simulink model "mainLinR2"  (R2017a)
settings: Solver=ode45  StartTime=0.0  StopTime=Tsim  RelTol=1e-3
values from neighbouring files (symbols this model uses):
  D = C2.Kd    [mainRun.m]
  F = -2    [mainRun.m]
  g = .5    (= 0.5)    [mainRun.m]
  Gamma = 10*eye(4)    [mainRun.m]
  I = C2.Ki    [mainRun.m]
  Kr0 = 0    [mainRun.m]
  Kx0 = 0    [mainRun.m]
  N = 2    [ident_wynik.m]    (also in mainRun.m = 1/C2.Tf; odp_czas.m = size(wyjscia,2); wykresyBode.m = length(modele))
  NAref = mrac.A    [mainRun.m]
  NBref = mrac.B    [mainRun.m]
  NCref = mrac.C    [mainRun.m]
  Nxref0 = zeros(2,1)    [mainRun.m]
  p0 = 1    [mainRun.m]
  phi0 = zeros(4,1)    [mainRun.m]
  PPid = C2.Kp    [mainRun.m]
  szum = 2e-4    (= 0.0002)    [mainRun.m]
  Th0 = zeros(4,1)    [mainRun.m]
  w10 = 0    [mainRun.m]
  w20 = 0    [mainRun.m]
  Xref0 = 0    [mainRun.m]
undefined symbols (not defined in the file or in its folder): GammaR, GammaX, P
libraries: bloki_pomocnicze x12, simulink x2, dspstat3 x2
settings Model: Creator=Piotr  LastModifiedBy=Piotr
settings SolverCC: ZeroCrossAlgorithm=Adaptive
settings OptimizationCC: EfficientFloat2IntCast=on
settings DebuggingCC: MaskedZcDiagnostic=none  IgnoredZcDiagnostic=none

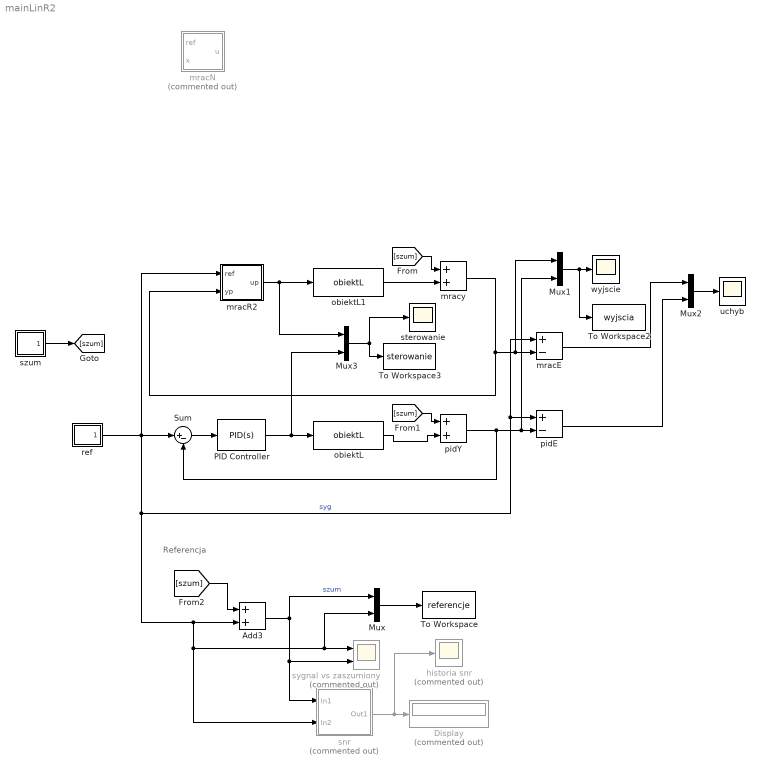
== system mainLinR2 ==
  note: Referencja
  Add3 : Sum
  Display : Display  Commented=on
  Mux{,1..3} (4 alike) : Mux  Inputs=2
  PID Controller : simulink/Continuous/PID Controller  Controller=PID  TimeDomain=Continuous-time  SampleTime=-1  IntegratorMethod=Forward Euler  FilterMethod=Forward Euler  Form=Parallel  UseFilter=on  ControllerParametersSource=internal  P=PPid  I=I  D=D  N=N  InitialConditionSource=internal  InitialConditionForIntegrator=0  InitialConditionForFilter=0  ExternalReset=none  LimitOutput=off  UpperSaturationLimit=1e6  LowerSaturationLimit=-1e6  LinearizeAsGain=on  AntiWindupMode=none  Kb=1  TrackingMode=off  Kt=1  PParamMin=[]  PParamMax=[]  IParamMin=[]  IParamMax=[]  DParamMin=[]  DParamMax=[]  NParamMin=[]  NParamMax=[]  KbParamMin=[]  KbParamMax=[]  KtParamMin=[]  KtParamMax=[]  POutMin=[]  POutMax=[]  IOutMin=[]  IOutMax=[]  DOutMin=[]  DOutMax=[]  NOutMin=[]  NOutMax=[]  KbOutMin=[]  KbOutMax=[]  KtOutMin=[]  KtOutMax=[]  IntegratorOutMin=[]  IntegratorOutMax=[]  FilterOutMin=[]  FilterOutMax=[]  SumOutMin=[]  SumOutMax=[]  SumI1OutMin=[]  SumI1OutMax=[]  SumI2OutMin=[]  SumI2OutMax=[]  SumI3OutMin=[]  SumI3OutMax=[]  SumDOutMin=[]  SumDOutMax=[]  SaturationOutMin=[]  SaturationOutMax=[]  IntegratorContinuousStateAttributes=''  IntegratorStateMustResolveToSignalObject=off  IntegratorRTWStateStorageClass=Auto  FilterContinuousStateAttributes=''  FilterStateMustResolveToSignalObject=off  FilterRTWStateStorageClass=Auto  DifferentiatorICPrevScaledInput=0  DifferentiatorOutMin=[]  DifferentiatorOutMax=[]  InitialConditionSetting=State (most efficient)
  Sum : Sum  Inputs=|+-
  To Workspace : ToWorkspace  VariableName=referencje  SampleTime=-1
  To Workspace2 : ToWorkspace  VariableName=wyjscia  SampleTime=-1
  To Workspace3 : ToWorkspace  VariableName=sterowanie  SampleTime=-1
  historia snr : Scope  Commented=on
  mracE : Sum  Inputs=+-
  mracN : Subsystem  Commented=on
  mracR2 : Subsystem  AncestorBlock=bloki_pomocnicze/mracR2
  mracy : Sum
  obiektL : bloki_pomocnicze/obiektL  SystemSampleTime=-1
  obiektL1 : bloki_pomocnicze/obiektL  SystemSampleTime=-1
  pidE : Sum  Inputs=+-
  pidY : Sum
  ref : Subsystem
  snr : Subsystem  Commented=on
  sterowanie : Scope
  sygnal vs zaszumiony : Scope  Commented=on  NumInputPorts=2
  szum : Subsystem
  uchyb : Scope
  wyjscie : Scope
  wires:
  PID Controller/1 -> Mux3/2, obiektL/1
  Sum/1 -> PID Controller/1
  pidY/1 -> Sum/2, Mux1/2, pidE/2
  mracy/1 -> mracR2/2(yp), Mux1/1, mracE/2
  mracE/1 -> Mux2/1
  pidE/1 -> Mux2/2
  Add3/1 -> snr/1(In1), sygnal vs zaszumiony/2, Mux/1  "szum"
  snr/1(Out1) -> historia snr/1, Display/1
  szum/1(Out1) -> [szum]
  obiektL1/1 -> mracy/2
  [szum] -> mracy/1
  obiektL/1 -> pidY/2
  [szum] -> pidY/1
  [szum] -> Add3/1
  ref/1(Out1) -> mracR2/1(ref), mracE/1, pidE/1, Add3/2, snr/2(In2), sygnal vs zaszumiony/1, Mux/2, Sum/1  "syg"
  Mux/1 -> To Workspace/1
  Mux1/1 -> To Workspace2/1, wyjscie/1
  Mux2/1 -> uchyb/1
  Mux3/1 -> To Workspace3/1, sterowanie/1
  mracR2/1(up) -> Mux3/1, obiektL1/1

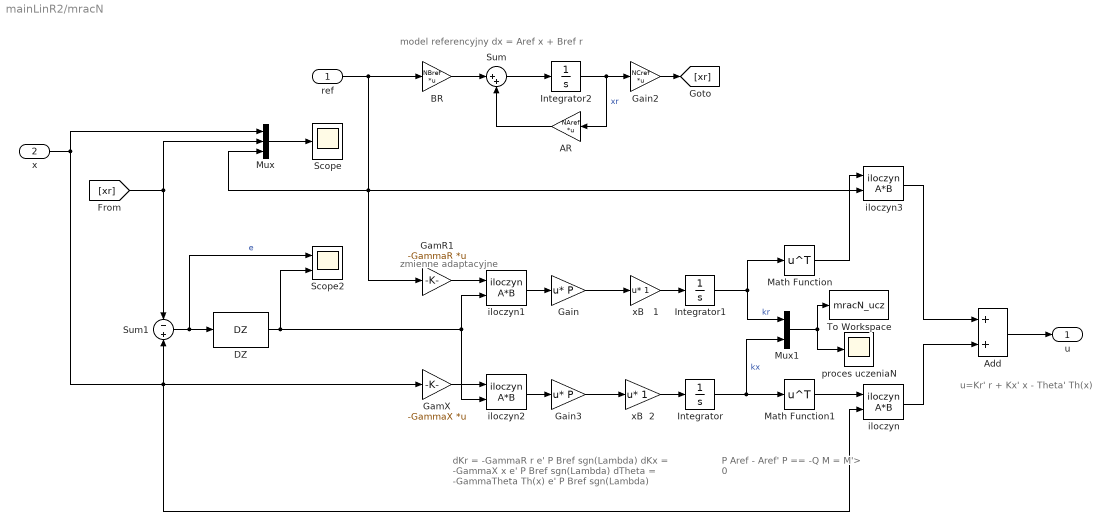
== system mainLinR2/mracN ==
  note: P Aref - Aref' P == -Q
      |
      | M = M'> 0
  note: dKr = -GammaR r e' P Bref sgn(Lambda)
      | dKx = -GammaX x e' P Bref sgn(Lambda)
      | dTheta = -GammaTheta Th(x) e' P Bref sgn(Lambda)
  note: zmienne adaptacyjne
  note: model referencyjny dx = Aref x + Bref r
  note: u=Kr' r + Kx' x - Theta' Th(x)
  ref : Inport
  x : Inport  Port=2
  AR : Gain  Gain=NAref  Multiplication=Matrix(K*u)
  Add : Sum
  BR : Gain  Gain=NBref  Multiplication=Matrix(K*u)
  DZ : bloki_pomocnicze/DZ  max=epsilonN
  Gain : Gain  Gain=P  Multiplication=Matrix(u*K)
  Gain2 : Gain  Gain=NCref  Multiplication=Matrix(K*u)
  Gain3 : Gain  Gain=P  Multiplication=Matrix(u*K)
  GamR1 : Gain  Gain=-GammaR  Multiplication=Matrix(K*u)
  GamX : Gain  Gain=-GammaX  Multiplication=Matrix(K*u)
  Integrator : Integrator  InitialCondition=Kx0
  Integrator1 : Integrator  InitialCondition=Kr0
  Integrator2 : Integrator  InitialCondition=Xref0
  Math Function : Math  Operator=transpose  SaturateOnIntegerOverflow=on
  Math Function1 : Math  Operator=transpose  SaturateOnIntegerOverflow=on
  Mux : Mux  Inputs=3
  Mux1 : Mux  Inputs=2
  Scope : Scope
  Scope2 : Scope  NumInputPorts=2
  Sum : Sum  Inputs=|++
  Sum1 : Sum  Inputs=-+
  To Workspace : ToWorkspace  VariableName=mracN_ucz  SampleTime=-1
  iloczyn{,1..3} (4 alike) : bloki_pomocnicze/iloczyn A*B  SystemSampleTime=-1
  proces uczeniaN : Scope
  xB   1 : Gain  Multiplication=Matrix(u*K)
  xB  2 : Gain  Multiplication=Matrix(u*K)
  u : Outport  PortDimensions=1
  wires:
  Add/1 -> u/1
  iloczyn/1 -> Add/2
  iloczyn1/1 -> Gain/1
  Integrator1/1 -> Mux1/1, Math Function/1  "kr"
  GamX/1 -> iloczyn2/1
  Gain/1 -> xB   1/1
  BR/1 -> Sum/1
  Integrator/1 -> Mux1/2, Math Function1/1  "kx"
  iloczyn3/1 -> Add/1
  Integrator2/1 -> AR/1, Gain2/1  "xr"
  Sum/1 -> Integrator2/1
  xB  2/1 -> Integrator/1
  AR/1 -> Sum/2
  Sum1/1 -> Scope2/1, DZ/1  "e"
  xB   1/1 -> Integrator1/1
  Gain3/1 -> xB  2/1
  GamR1/1 -> iloczyn1/1
  iloczyn2/1 -> Gain3/1
  Math Function/1 -> iloczyn3/1
  [xr] -> Mux/2, Sum1/1
  Math Function1/1 -> iloczyn/1
  Gain2/1 -> [xr]
  x/1 -> iloczyn/2, Sum1/2, GamX/1, Mux/1
  Mux/1 -> Scope/1
  DZ/1 -> iloczyn1/2, iloczyn2/2, Scope2/2
  ref/1 -> Mux/3, GamR1/1, iloczyn3/2, BR/1
  Mux1/1 -> proces uczeniaN/1, To Workspace/1

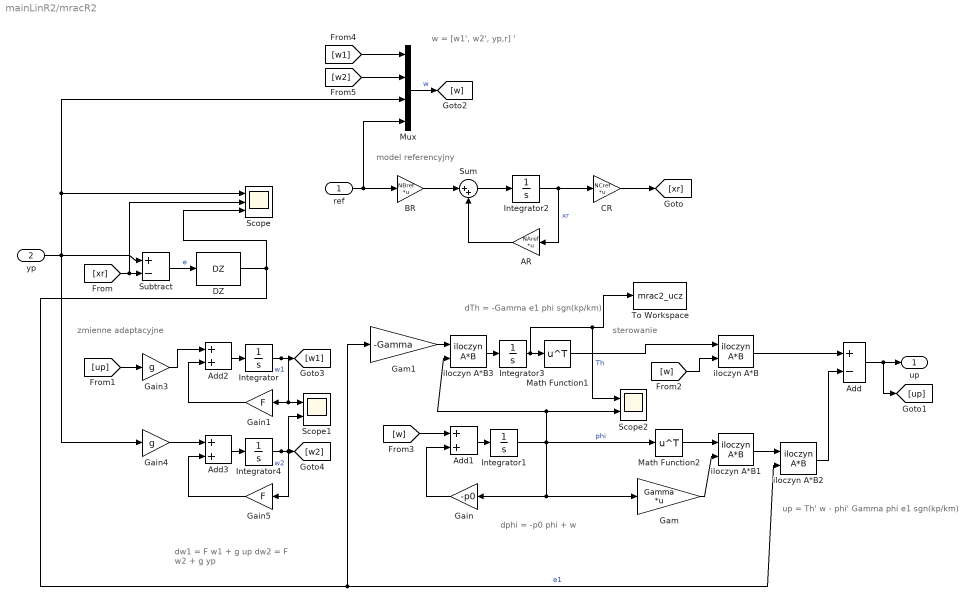
== system mainLinR2/mracR2 ==
  note: up = Th' w - phi' Gamma phi e1 sgn(kp/km)
  note: model referencyjny
  note: zmienne adaptacyjne
  note: dw1 = F w1 + g up
      |
      | dw2 = F w2 + g yp
  note: dTh = -Gamma e1 phi sgn(kp/km)
  note: dphi = -p0 phi + w
  note: w = [w1', w2', yp,r] '
  note: sterowanie
  ref : Inport
  yp : Inport  Port=2
  AR : Gain  Gain=NAref  Multiplication=Matrix(K*u)
  Add : Sum  Inputs=+-
  Add1 : Sum
  Add2 : Sum
  Add3 : Sum
  BR : Gain  Gain=NBref  Multiplication=Matrix(K*u)
  CR : Gain  Gain=NCref  Multiplication=Matrix(K*u)
  DZ : bloki_pomocnicze/DZ  max=epsilon2
  Gain : Gain  Gain=-p0
  Gain1 : Gain  Gain=F
  Gain3 : Gain  Gain=g
  Gain4 : Gain  Gain=g
  Gain5 : Gain  Gain=F
  Gam : Gain  Gain=Gamma  Multiplication=Matrix(K*u)
  Gam1 : Gain  Gain=-Gamma
  Integrator : Integrator  InitialCondition=w10
  Integrator1 : Integrator  InitialCondition=phi0
  Integrator2 : Integrator  InitialCondition=Nxref0
  Integrator3 : Integrator  InitialCondition=Th0
  Integrator4 : Integrator  InitialCondition=w20
  Math Function1 : Math  Operator=transpose  SaturateOnIntegerOverflow=on
  Math Function2 : Math  Operator=transpose  SaturateOnIntegerOverflow=on
  Mux : Mux
  Scope : Scope  NumInputPorts=3
  Scope1 : Scope  NumInputPorts=2
  Scope2 : Scope  NumInputPorts=2
  Subtract : Sum  Inputs=+-
  Sum : Sum  Inputs=|++
  To Workspace : ToWorkspace  VariableName=mrac2_ucz  SampleTime=-1
  iloczyn A*B{,1..3} (4 alike) : bloki_pomocnicze/iloczyn A*B  SystemSampleTime=-1
  up : Outport
  wires:
  iloczyn A*B3/1 -> Integrator3/1
  [w2] -> Mux/2
  [w1] -> Mux/1
  [w] -> Add1/1
  Add3/1 -> Integrator4/1
  Integrator4/1 -> [w2], Scope1/2, Gain5/1  "w2"
  Gain5/1 -> Add3/2
  Gain4/1 -> Add3/1
  Gain3/1 -> Add2/1
  [up] -> Gain3/1
  Gain1/1 -> Add2/2
  Integrator/1 -> [w1], Scope1/1, Gain1/1  "w1"
  Gam1/1 -> iloczyn A*B3/1
  iloczyn A*B2/1 -> Add/2
  iloczyn A*B1/1 -> iloczyn A*B2/1
  Gam/1 -> iloczyn A*B1/2
  Math Function2/1 -> iloczyn A*B1/1
  Mux/1 -> [w]  "w"
  Integrator3/1 -> To Workspace/1, Scope2/1, Math Function1/1  "Th"
  Gain/1 -> Add1/2
  Add1/1 -> Integrator1/1
  DZ/1 -> Scope/3, iloczyn A*B2/2, Gam1/1  "e1"
  Subtract/1 -> DZ/1  "e"
  ref/1 -> Mux/4, BR/1
  yp/1 -> Gain4/1, Subtract/1, Mux/3, Scope/1
  [xr] -> Scope/2, Subtract/2
  AR/1 -> Sum/2
  Add2/1 -> Integrator/1
  Sum/1 -> Integrator2/1
  Integrator2/1 -> AR/1, CR/1  "xr"
  BR/1 -> Sum/1
  Integrator1/1 -> iloczyn A*B3/2, Scope2/2, Gain/1, Gam/1, Math Function2/1  "phi"
  Add/1 -> up/1, [up]
  CR/1 -> [xr]
  Math Function1/1 -> iloczyn A*B/1
  [w] -> iloczyn A*B/2
  iloczyn A*B/1 -> Add/1

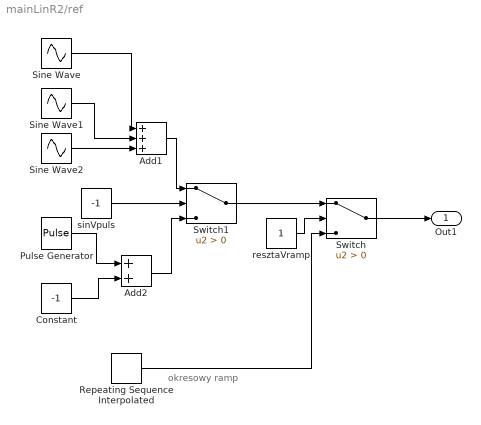
== system mainLinR2/ref ==
  note: okresowy ramp
  Add1 : Sum  Inputs=+++
  Add2 : Sum
  Constant : Constant  Value=-1
  Pulse Generator : DiscretePulseGenerator  PulseType=Time based  Amplitude=2  Period=20  PulseWidth=50
  Repeating Sequence Interpolated : simulink/Sources/Repeating Sequence Interpolated  OutValues=[0 1 1 0 -1 -1 0].'*10  TimeValues=cumsum([0 1e-2 0.7 0.1 0.1 0.7 0.7]).'*12  LookUpMeth=Interpolation-Use End Values  tsamp=0.01  OutMin=[]  OutMax=[]  OutDataTypeStr=double  OutputDataTypeScalingMode=double  OutDataType=fixdt(0,8)  OutScaling=2^-10
  Sine Wave : Sin  Amplitude=25  Frequency=0.3  SampleTime=0
  Sine Wave1 : Sin  Amplitude=2  Frequency=2  SampleTime=0
  Sine Wave2 : Sin  Amplitude=10  Frequency=0.4  Phase=0.5  SampleTime=0
  Switch : Switch  Criteria=u2 > Threshold
  Switch1 : Switch  Criteria=u2 > Threshold
  resztaVramp : Constant
  sinVpuls : Constant  Value=-1
  Out1 : Outport
  wires:
  Switch/1 -> Out1/1
  Constant/1 -> Add2/2
  Pulse Generator/1 -> Add2/1
  Repeating Sequence Interpolated/1 -> Switch/3
  Sine Wave/1 -> Add1/1
  resztaVramp/1 -> Switch/2
  sinVpuls/1 -> Switch1/2
  Switch1/1 -> Switch/1
  Add2/1 -> Switch1/3
  Add1/1 -> Switch1/1
  Sine Wave1/1 -> Add1/2
  Sine Wave2/1 -> Add1/3

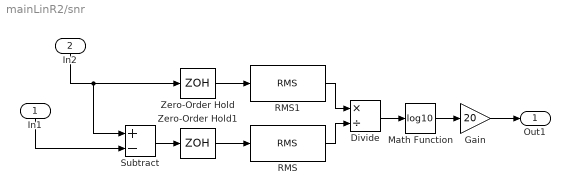
== system mainLinR2/snr ==
  In1 : Inport
  In2 : Inport  Port=2
  Divide : Product  Inputs=*/
  Gain : Gain  Gain=20
  Math Function : Math  Operator=log10  SaturateOnIntegerOverflow=on
  RMS : dspstat3/RMS  run=on  directionMode=Each column  dimension=1  InputProcessing=Columns as channels (frame based)  reset_popup=None
  RMS1 : dspstat3/RMS  run=on  directionMode=Each column  dimension=1  InputProcessing=Columns as channels (frame based)  reset_popup=None
  Subtract : Sum  Inputs=+-
  Zero-Order Hold : ZeroOrderHold  SampleTime=-1
  Zero-Order Hold1 : ZeroOrderHold  SampleTime=-1
  Out1 : Outport
  wires:
  Gain/1 -> Out1/1
  Divide/1 -> Math Function/1
  RMS/1 -> Divide/2
  Math Function/1 -> Gain/1
  RMS1/1 -> Divide/1
  In1/1 -> Subtract/2
  In2/1 -> Zero-Order Hold/1, Subtract/1
  Zero-Order Hold/1 -> RMS1/1
  Zero-Order Hold1/1 -> RMS/1
  Subtract/1 -> Zero-Order Hold1/1

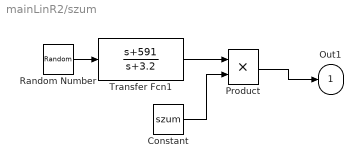
== system mainLinR2/szum ==
  Constant : Constant  Value=szum
  Product : Product
  Random Number : RandomNumber  SampleTime=0.1
  Transfer Fcn1 : TransferFcn  Numerator=[1 591]  Denominator=[1 3.2]
  Out1 : Outport
  wires:
  Product/1 -> Out1/1
  Transfer Fcn1/1 -> Product/1
  Random Number/1 -> Transfer Fcn1/1
  Constant/1 -> Product/2
